simulink model "nn_fuel_control_4_15"  (R2021a)
settings: Solver=ode15s  StartTime=0.0  StopTime=T  MaxStep=.01  RelTol=1e-3
undefined symbols (not defined in the file): AF_sensor_tol, fault_time, fuel_inj_tol, kappa_tol, MAF_sensor_tol, pump_tol, tau_ww_tol
libraries: neural x66
(part 3 of 3)

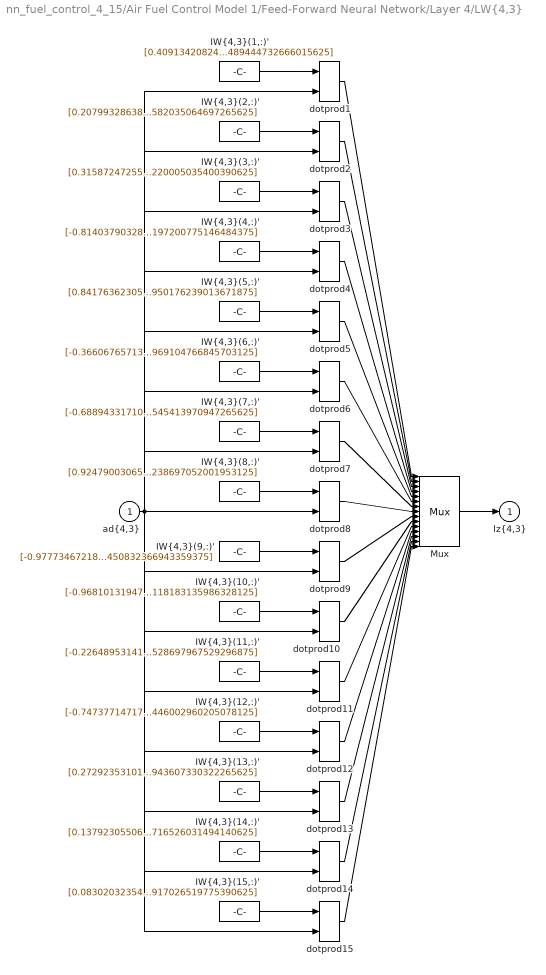
== system nn_fuel_control_4_15/Air Fuel Control Model 1/Feed-Forward Neural Network/Layer 4/LW{4,3} ==
  "ad{4,3}" : Inport  PortDimensions=15
      mask Display: e = 0.06;c1 = [120 230 180]/255;c2 = ([120 230 180]+0)/(256+128);c3 = ([120 230 180]+128)/(256+128);patch([0 1 1 0],[0 0 1 1],c1);patch([0 1 1 1-e 1-e 0+e],[0 0 1 1-e 0+e 0+e],c2);patch([0 0 1 1-e 0+e 0+e],[0 1 1 1-e 1-e 0+e],c3);plot([0 1 1 0 0],[0 0 1 1 0]);
  "IW{4,3}(1,:)'" : Constant  Value=[0.409134208241364427660613500847830437123775482177734375;-0.018608604712277689030575089645935804583132266998291015625;-0.429419328749681750156952375618857331573963165283203125;0.0968634595111320939597732149195508100092411041259765625;0.161200991521329939359929994679987430572509765625;-0.008332083953835521528130669821621268056333065032958984375;0.2000331787879461586943108386549283750355243682861328125;0.10950567443581950277664560644552693702280521392822265625;0.2065467508985891764705655759826186113059520721435546875;0.9045530959878378407523769055842421948909759521484375;0.0283070330066618157383029341644942178390920162200927734375;0.1527128132980928310047374907298944890499114990234375;0.57805498370952645981191153623512946069240570068359375;-0.493604151024888526677614208892919123172760009765625;0.29996514325046830240495410180301405489444732666015625]
      mask Display: e = 0.06;c1 = [120 150 230]/255;c2 = ([120 150 230]+0)/383;c3 = ([120 150 230]+128)/383;patch([0 1 1 0],[0 0 1 1],c1);patch([0 1 1 1-e 1-e 0+e],[0 0 1 1-e 0+e 0+e],c2);patch([0 0 1 1-e 0+e 0+e],[0 1 1 1-e 1-e 0+e],c3);plot([0 1 1 0 0],[0 0 1 1 0]);disp('weights');
  "IW{4,3}(10,:)'" : Constant  Value=[-0.9681013194700429647099326757597737014293670654296875;0.308531151003858639114696416072547435760498046875;0.5238840389262133800940546279889531433582305908203125;-0.8084989587128526000725514677469618618488311767578125;-0.801873444424249459672182638314552605152130126953125;0.142650764746548308625762047086027450859546661376953125;-0.63857819911989810446328874604660086333751678466796875;-0.174290199895392905471425137875485233962535858154296875;-0.34415160909336417471848790228250436484813690185546875;-0.6047578233492736377030496441875584423542022705078125;-0.5627993624805025518753609503619372844696044921875;0.2576274618067879718097401564591564238071441650390625;-0.12046847177087678659734848451989819295704364776611328125;0.7481637664193332426521010347642004489898681640625;0.71881850459924578888859514336218126118183135986328125]
      mask Display: e = 0.06;c1 = [120 150 230]/255;c2 = ([120 150 230]+0)/383;c3 = ([120 150 230]+128)/383;patch([0 1 1 0],[0 0 1 1],c1);patch([0 1 1 1-e 1-e 0+e],[0 0 1 1-e 0+e 0+e],c2);patch([0 0 1 1-e 0+e 0+e],[0 1 1 1-e 1-e 0+e],c3);plot([0 1 1 0 0],[0 0 1 1 0]);disp('weights');
  "IW{4,3}(11,:)'" : Constant  Value=[-0.22648953141163108426781036541797220706939697265625;-0.4126513309446071531283450894989073276519775390625;-0.919897514578432495824245052062906324863433837890625;-0.4049584327914892423194714865530841052532196044921875;-0.9260658560814845063902112087816931307315826416015625;0.247532816868120786324425353086553514003753662109375;-0.8130784976056506518915512060630135238170623779296875;-0.1161494390508523988359002032666467130184173583984375;0.76460872230926124615280059515498578548431396484375;0.530450464187323778020299869240261614322662353515625;-0.6035021468768022590012378714163787662982940673828125;0.0287139365740867180676332282018847763538360595703125;-0.2066484644619717148117388205719180405139923095703125;-0.5723818088758767519408365842537023127079010009765625;-0.5211382354194913357758878191816620528697967529296875]
      mask Display: e = 0.06;c1 = [120 150 230]/255;c2 = ([120 150 230]+0)/383;c3 = ([120 150 230]+128)/383;patch([0 1 1 0],[0 0 1 1],c1);patch([0 1 1 1-e 1-e 0+e],[0 0 1 1-e 0+e 0+e],c2);patch([0 0 1 1-e 0+e 0+e],[0 1 1 1-e 1-e 0+e],c3);plot([0 1 1 0 0],[0 0 1 1 0]);disp('weights');
  "IW{4,3}(12,:)'" : Constant  Value=[-0.747377147172722633428065819316543638706207275390625;-0.89961393161859748435205119676538743078708648681640625;-0.037086697665867023043784200808659079484641551971435546875;-0.5886496554696816208007703608018346130847930908203125;0.840702237392853657382829624111764132976531982421875;0.68778578029264991755553637631237506866455078125;-0.09030666083632643559298003310686908662319183349609375;0.5165108873683141865740253706462681293487548828125;-0.89460884910017035576146327002788893878459930419921875;-0.82058175976433034293222590349614620208740234375;0.6131893427537697949247785800253041088581085205078125;0.699855135033757402851506412844173610210418701171875;-0.335585846707859014603769765017204917967319488525390625;0.0423943456344091362808512712945230305194854736328125;0.297963040188151062626076281958376057446002960205078125]
      mask Display: e = 0.06;c1 = [120 150 230]/255;c2 = ([120 150 230]+0)/383;c3 = ([120 150 230]+128)/383;patch([0 1 1 0],[0 0 1 1],c1);patch([0 1 1 1-e 1-e 0+e],[0 0 1 1-e 0+e 0+e],c2);patch([0 0 1 1-e 0+e 0+e],[0 1 1 1-e 1-e 0+e],c3);plot([0 1 1 0 0],[0 0 1 1 0]);disp('weights');
  "IW{4,3}(13,:)'" : Constant  Value=[0.27292353101536026560580694422242231667041778564453125;0.291784885724885867386291238290141336619853973388671875;0.8796340464296978911562518987921066582202911376953125;0.307061729491277357606549003321561031043529510498046875;-0.3222728751950858505637143025523982942104339599609375;0.0304681963646269045320469359694470767863094806671142578125;-0.2456543422635725504310499900384456850588321685791015625;-0.89682596908113521028127479439717717468738555908203125;-0.28255076861598527049324047766276635229587554931640625;0.3030535285194508876571717337355948984622955322265625;-0.67415060674015503394684856175445020198822021484375;0.6670352766341516304038350426708348095417022705078125;0.2667146340046648855803823607857339084148406982421875;-0.045954538378264686571128549985587596893310546875;0.2340639218102315288749792898670420981943607330322265625]
      mask Display: e = 0.06;c1 = [120 150 230]/255;c2 = ([120 150 230]+0)/383;c3 = ([120 150 230]+128)/383;patch([0 1 1 0],[0 0 1 1],c1);patch([0 1 1 1-e 1-e 0+e],[0 0 1 1-e 0+e 0+e],c2);patch([0 0 1 1-e 0+e 0+e],[0 1 1 1-e 1-e 0+e],c3);plot([0 1 1 0 0],[0 0 1 1 0]);disp('weights');
  "IW{4,3}(14,:)'" : Constant  Value=[0.1379230550644596764442439962294884026050567626953125;0.4775263823187978484696714076562784612178802490234375;-0.006364787120916037821416466613300144672393798828125;0.43980447972305025672312694950960576534271240234375;-0.6384608804287079664163684356026351451873779296875;-0.03130848387336104821088156313635408878326416015625;0.9574895373112684016092543970444239675998687744140625;-0.0896234843262868619007122106268070638179779052734375;0.1527953241303305897957898196182213723659515380859375;-0.1292468261657202521774934211862273514270782470703125;-0.970451720093115977050501896883361041545867919921875;-0.165062170367600291598364492529071867465972900390625;-0.7332719341796412049205855510081164538860321044921875;0.15986676798598864479572512209415435791015625;-0.6782299146816017643146778937079943716526031494140625]
      mask Display: e = 0.06;c1 = [120 150 230]/255;c2 = ([120 150 230]+0)/383;c3 = ([120 150 230]+128)/383;patch([0 1 1 0],[0 0 1 1],c1);patch([0 1 1 1-e 1-e 0+e],[0 0 1 1-e 0+e 0+e],c2);patch([0 0 1 1-e 0+e 0+e],[0 1 1 1-e 1-e 0+e],c3);plot([0 1 1 0 0],[0 0 1 1 0]);disp('weights');
  "IW{4,3}(15,:)'" : Constant  Value=[0.08302032354421218229845180758275091648101806640625;0.249954151496840193402704244363121688365936279296875;0.5479301525869659794665267327218316495418548583984375;0.1693125052219013326748608960770070552825927734375;0.7569645787080911958355500246398150920867919921875;-0.8852503867351309008171256209607236087322235107421875;-0.6961185761680448447208391371532343327999114990234375;-0.5600757389611796810413579805754125118255615234375;-0.0720835330077151947847369228838942945003509521484375;0.855447974963159385453081995365209877490997314453125;0.167257696778575937202049317420460283756256103515625;-0.2562635879714936226747568071004934608936309814453125;-0.90062487978110539188492111861705780029296875;-0.11820475372601801922201048000715672969818115234375;-0.4539894984214323248039590907865203917026519775390625]
      mask Display: e = 0.06;c1 = [120 150 230]/255;c2 = ([120 150 230]+0)/383;c3 = ([120 150 230]+128)/383;patch([0 1 1 0],[0 0 1 1],c1);patch([0 1 1 1-e 1-e 0+e],[0 0 1 1-e 0+e 0+e],c2);patch([0 0 1 1-e 0+e 0+e],[0 1 1 1-e 1-e 0+e],c3);plot([0 1 1 0 0],[0 0 1 1 0]);disp('weights');
  "IW{4,3}(2,:)'" : Constant  Value=[0.2079932863873300286083889432120486162602901458740234375;0.0198375850467484675376805824953407864086329936981201171875;-0.0170538332699734680730774272205962915904819965362548828125;-0.78563968744001211330640899177524261176586151123046875;-0.2368930020652066925634926519705913960933685302734375;0.9350198499073567592887457067263312637805938720703125;-0.12408787305239055154260086055728606879711151123046875;0.405654658867162176694165509616141207516193389892578125;0.53267120540349510715572023400454781949520111083984375;0.2861429337433631925335930645815096795558929443359375;0.55828534790967221379531792990746907889842987060546875;0.1589999460246069862279227891121990978717803955078125;-0.67481637945571459891169752154382877051830291748046875;0.1334057042983116669887522220960818231105804443359375;0.7580972863172894538053014912293292582035064697265625]
      mask Display: e = 0.06;c1 = [120 150 230]/255;c2 = ([120 150 230]+0)/383;c3 = ([120 150 230]+128)/383;patch([0 1 1 0],[0 0 1 1],c1);patch([0 1 1 1-e 1-e 0+e],[0 0 1 1-e 0+e 0+e],c2);patch([0 0 1 1-e 0+e 0+e],[0 1 1 1-e 1-e 0+e],c3);plot([0 1 1 0 0],[0 0 1 1 0]);disp('weights');
  "IW{4,3}(3,:)'" : Constant  Value=[0.315872472556143424338159775288659147918224334716796875;0.1333374680748961316201217641719267703592777252197265625;-0.8918022391931847980828251820639707148075103759765625;0.7229899645184658663055188299040310084819793701171875;-0.2253949295409380937371679465286433696746826171875;0.43626032290268312863190658390522003173828125;-0.328908135182625349646201584619120694696903228759765625;-0.458606144094257428545091670457622967660427093505859375;-0.61397105979310195866816002308041788637638092041015625;0.687755868493051369938484640442766249179840087890625;-0.55032022765885801884877537304419092833995819091796875;-0.984145967069915972302851514541544020175933837890625;0.659406042092762323392207690631039440631866455078125;0.7727829791426754635352835975936613976955413818359375;-0.2628597007919442063439419143833220005035400390625]
      mask Display: e = 0.06;c1 = [120 150 230]/255;c2 = ([120 150 230]+0)/383;c3 = ([120 150 230]+128)/383;patch([0 1 1 0],[0 0 1 1],c1);patch([0 1 1 1-e 1-e 0+e],[0 0 1 1-e 0+e 0+e],c2);patch([0 0 1 1-e 0+e 0+e],[0 1 1 1-e 1-e 0+e],c3);plot([0 1 1 0 0],[0 0 1 1 0]);disp('weights');
  "IW{4,3}(4,:)'" : Constant  Value=[-0.814037903285731001545855178846977651119232177734375;0.1890950378764437445067159160316805355250835418701171875;0.136401296266547567004323582295910455286502838134765625;0.360474784994809394067516450377297587692737579345703125;0.5630045830298939790736767463386058807373046875;0.29464287473444394915844668503268621861934661865234375;-0.166389331488835556793759451466030441224575042724609375;-0.52974791348181538008788038496277295053005218505859375;0.6709267757531172104989991566981188952922821044921875;0.78215070403519337816078405012376606464385986328125;-0.3475888728410432282345254861866123974323272705078125;-0.05233329279450771309711853973567485809326171875;-0.30839028431399395646650418711942620575428009033203125;-0.7896972970706410688279675014200620353221893310546875;-0.17608840795251889943529022275470197200775146484375]
      mask Display: e = 0.06;c1 = [120 150 230]/255;c2 = ([120 150 230]+0)/383;c3 = ([120 150 230]+128)/383;patch([0 1 1 0],[0 0 1 1],c1);patch([0 1 1 1-e 1-e 0+e],[0 0 1 1-e 0+e 0+e],c2);patch([0 0 1 1-e 0+e 0+e],[0 1 1 1-e 1-e 0+e],c3);plot([0 1 1 0 0],[0 0 1 1 0]);disp('weights');
  "IW{4,3}(5,:)'" : Constant  Value=[0.84176362305803476004939511767588555812835693359375;0.2477725819719711619626423271256498992443084716796875;0.5861173758530409116929149604402482509613037109375;-0.2752688473484992126572024062625132501125335693359375;0.51232493805437240297351308981887996196746826171875;-0.617883791172630925103703702916391193866729736328125;0.0601814606396653406505947714322246611118316650390625;-0.407352526024439942631261146743781864643096923828125;-0.2072883860196756966587372517096810042858123779296875;-0.49975965526174181974283783347345888614654541015625;-0.40148233621736295617665746249258518218994140625;-0.852800606242346770358153662527911365032196044921875;-0.9196593002841557673576744491583667695522308349609375;0.2861473976537853847190717715420760214328765869140625;-0.1468670488112422400917012055288068950176239013671875]
      mask Display: e = 0.06;c1 = [120 150 230]/255;c2 = ([120 150 230]+0)/383;c3 = ([120 150 230]+128)/383;patch([0 1 1 0],[0 0 1 1],c1);patch([0 1 1 1-e 1-e 0+e],[0 0 1 1-e 0+e 0+e],c2);patch([0 0 1 1-e 0+e 0+e],[0 1 1 1-e 1-e 0+e],c3);plot([0 1 1 0 0],[0 0 1 1 0]);disp('weights');
  "IW{4,3}(6,:)'" : Constant  Value=[-0.366067657130750567784360782752628438174724578857421875;-0.5885259561877165257470778669812716543674468994140625;-0.73842489905764419066969139748835004866123199462890625;0.714576283962894631685003332677297294139862060546875;-0.0609476018705905620009843914886005222797393798828125;0.73355928402501680007929962812340818345546722412109375;0.1474523444056059506834799321950413286685943603515625;-0.2160830186712152656269836370483972132205963134765625;0.33658785604271823643784955493174493312835693359375;-0.6737160690455079592453557779663242399692535400390625;0.49385592210495332654573985564638860523700714111328125;-0.6063479899954280494256408928777091205120086669921875;0.6470220483020143742436403044848702847957611083984375;-0.205829216943276716023092376417480409145355224609375;-0.920350237519944158748330664820969104766845703125]
      mask Display: e = 0.06;c1 = [120 150 230]/255;c2 = ([120 150 230]+0)/383;c3 = ([120 150 230]+128)/383;patch([0 1 1 0],[0 0 1 1],c1);patch([0 1 1 1-e 1-e 0+e],[0 0 1 1-e 0+e 0+e],c2);patch([0 0 1 1-e 0+e 0+e],[0 1 1 1-e 1-e 0+e],c3);plot([0 1 1 0 0],[0 0 1 1 0]);disp('weights');
  "IW{4,3}(7,:)'" : Constant  Value=[-0.688943317105236818775892970734275877475738525390625;-0.5417308519282884038403835802455432713031768798828125;-0.2521322205228260227016789940535090863704681396484375;0.94374276814532809254387757391668856143951416015625;0.1889533323761056760048404612462036311626434326171875;-0.9318119687351316127177369708078913390636444091796875;0.4540745589147954230924142393632791936397552490234375;-0.5142256715696016389216538300388492643833160400390625;0.4877526756618586478708721188013441860675811767578125;-0.2884862767777562897464349589427001774311065673828125;0.3008932019526311396617757054627873003482818603515625;-0.089609771299732354776779175153933465480804443359375;0.5886547451838171074456340647884644567966461181640625;0.0935276670241786955983798179659061133861541748046875;-0.916953528583667409890267663286067545413970947265625]
      mask Display: e = 0.06;c1 = [120 150 230]/255;c2 = ([120 150 230]+0)/383;c3 = ([120 150 230]+128)/383;patch([0 1 1 0],[0 0 1 1],c1);patch([0 1 1 1-e 1-e 0+e],[0 0 1 1-e 0+e 0+e],c2);patch([0 0 1 1-e 0+e 0+e],[0 1 1 1-e 1-e 0+e],c3);plot([0 1 1 0 0],[0 0 1 1 0]);disp('weights');
  "IW{4,3}(8,:)'" : Constant  Value=[0.9247900306516465551709416104131378233432769775390625;-0.451872576203322662280470467521809041500091552734375;0.2144636938109696633336653803780791349709033966064453125;0.47393632788181161430429710890166461467742919921875;-0.5967841378403215824022254309966228902339935302734375;0.08921929855929823516280663397992611862719058990478515625;0.50281570056286717385063411711598746478557586669921875;-0.2361795031497051222668659420378389768302440643310546875;0.28420950093741248476675309575512073934078216552734375;-0.0425352900120927746030474736471660435199737548828125;0.393770417536720263029792477027513086795806884765625;0.6773406762422686799851589967147447168827056884765625;0.62704069904055137474330194891081191599369049072265625;0.0260862162785266971098963040276430547237396240234375;0.71691198886489904129604155968991108238697052001953125]
      mask Display: e = 0.06;c1 = [120 150 230]/255;c2 = ([120 150 230]+0)/383;c3 = ([120 150 230]+128)/383;patch([0 1 1 0],[0 0 1 1],c1);patch([0 1 1 1-e 1-e 0+e],[0 0 1 1-e 0+e 0+e],c2);patch([0 0 1 1-e 0+e 0+e],[0 1 1 1-e 1-e 0+e],c3);plot([0 1 1 0 0],[0 0 1 1 0]);disp('weights');
  "IW{4,3}(9,:)'" : Constant  Value=[-0.9777346721832860243495133545366115868091583251953125;0.3448850057379984068717249101609922945499420166015625;0.3117068047075581826987900058156810700893402099609375;-0.2800738720389521763109996754792518913745880126953125;0.1829551461951293145347108293208293616771697998046875;-0.036462488845966589678937452845275402069091796875;0.61637847324658689984744341927580535411834716796875;-0.97795607139009721464617541641928255558013916015625;-0.306381255697655507930221574497409164905548095703125;-0.3682386527599306180746907557477243244647979736328125;0.636545889474316783918084183824248611927032470703125;0.67733149686665061750545646646060049533843994140625;-0.1690740091796387734035533867427147924900054931640625;0.3344301037607857463029858990921638906002044677734375;-0.21065411005500944696677834144793450832366943359375]
      mask Display: e = 0.06;c1 = [120 150 230]/255;c2 = ([120 150 230]+0)/383;c3 = ([120 150 230]+128)/383;patch([0 1 1 0],[0 0 1 1],c1);patch([0 1 1 1-e 1-e 0+e],[0 0 1 1-e 0+e 0+e],c2);patch([0 0 1 1-e 0+e 0+e],[0 1 1 1-e 1-e 0+e],c3);plot([0 1 1 0 0],[0 0 1 1 0]);disp('weights');
  Mux : Mux  Inputs=15
      mask Display: e = 0.06;c1 = [120 150 230]/255;c2 = ([120 150 230]+0)/383;c3 = ([120 150 230]+128)/383;patch([0 1 1 0],[0 0 1 1],c1);patch([0 1 1 1-e 1-e 0+e],[0 0 1 1-e 0+e 0+e],c2);patch([0 0 1 1-e 0+e 0+e],[0 1 1 1-e 1-e 0+e],c3);plot([0 1 1 0 0],[0 0 1 1 0]);disp('Mux');
  dotprod{1..15} (15 alike) : neural/Weight Functions/dotprod
  "lz{4,3}" : Outport
      mask Display: e = 0.06;c1 = [120 230 180]/255;c2 = ([120 230 180]+0)/(256+128);c3 = ([120 230 180]+128)/(256+128);patch([0 1 1 0],[0 0 1 1],c1);patch([0 1 1 1-e 1-e 0+e],[0 0 1 1-e 0+e 0+e],c2);patch([0 0 1 1-e 0+e 0+e],[0 1 1 1-e 1-e 0+e],c3);plot([0 1 1 0 0],[0 0 1 1 0]);
  wires:
  "IW{4,3}(1,:)'"/1 -> dotprod1/1
  "ad{4,3}"/1 -> dotprod1/2, dotprod2/2, dotprod3/2, dotprod4/2, dotprod5/2, dotprod6/2, dotprod7/2, dotprod8/2, dotprod9/2, dotprod10/2, dotprod11/2, dotprod12/2, dotprod13/2, dotprod14/2, dotprod15/2
  dotprod1/1 -> Mux/1
  "IW{4,3}(2,:)'"/1 -> dotprod2/1
  dotprod2/1 -> Mux/2
  "IW{4,3}(3,:)'"/1 -> dotprod3/1
  dotprod3/1 -> Mux/3
  "IW{4,3}(4,:)'"/1 -> dotprod4/1
  dotprod4/1 -> Mux/4
  "IW{4,3}(5,:)'"/1 -> dotprod5/1
  dotprod5/1 -> Mux/5
  "IW{4,3}(6,:)'"/1 -> dotprod6/1
  dotprod6/1 -> Mux/6
  "IW{4,3}(7,:)'"/1 -> dotprod7/1
  dotprod7/1 -> Mux/7
  "IW{4,3}(8,:)'"/1 -> dotprod8/1
  dotprod8/1 -> Mux/8
  "IW{4,3}(9,:)'"/1 -> dotprod9/1
  dotprod9/1 -> Mux/9
  "IW{4,3}(10,:)'"/1 -> dotprod10/1
  dotprod10/1 -> Mux/10
  "IW{4,3}(11,:)'"/1 -> dotprod11/1
  dotprod11/1 -> Mux/11
  "IW{4,3}(12,:)'"/1 -> dotprod12/1
  dotprod12/1 -> Mux/12
  "IW{4,3}(13,:)'"/1 -> dotprod13/1
  dotprod13/1 -> Mux/13
  "IW{4,3}(14,:)'"/1 -> dotprod14/1
  dotprod14/1 -> Mux/14
  "IW{4,3}(15,:)'"/1 -> dotprod15/1
  dotprod15/1 -> Mux/15
  Mux/1 -> "lz{4,3}"/1

== system nn_fuel_control_4_15/Air Fuel Control Model 1/Feed-Forward Neural Network/Layer 5/Delays 1 ==
  "p{5}" : Inport  PortDimensions=15
      mask Display: e = 0.06;c1 = [120 230 180]/255;c2 = ([120 230 180]+0)/(256+128);c3 = ([120 230 180]+128)/(256+128);patch([0 1 1 0],[0 0 1 1],c1);patch([0 1 1 1-e 1-e 0+e],[0 0 1 1-e 0+e 0+e],c2);patch([0 0 1 1-e 0+e 0+e],[0 1 1 1-e 1-e 0+e],c3);plot([0 1 1 0 0],[0 0 1 1 0]);
  mux : Mux  Inputs=1
      mask Display: e = 0.06;c1 = [120 150 230]/255;c2 = ([120 150 230]+0)/383;c3 = ([120 150 230]+128)/383;patch([0 1 1 0],[0 0 1 1],c1);patch([0 1 1 1-e 1-e 0+e],[0 0 1 1-e 0+e 0+e],c2);patch([0 0 1 1-e 0+e 0+e],[0 1 1 1-e 1-e 0+e],c3);plot([0 1 1 0 0],[0 0 1 1 0]);disp('Mux')
  "pd{5,4}" : Outport
      mask Display: e = 0.06;c1 = [120 230 180]/255;c2 = ([120 230 180]+0)/(256+128);c3 = ([120 230 180]+128)/(256+128);patch([0 1 1 0],[0 0 1 1],c1);patch([0 1 1 1-e 1-e 0+e],[0 0 1 1-e 0+e 0+e],c2);patch([0 0 1 1-e 0+e 0+e],[0 1 1 1-e 1-e 0+e],c3);plot([0 1 1 0 0],[0 0 1 1 0]);
  wires:
  "p{5}"/1 -> mux/1
  mux/1 -> "pd{5,4}"/1

== system nn_fuel_control_4_15/Air Fuel Control Model 1/Feed-Forward Neural Network/Layer 5/LW{5,4} ==
  "ad{5,4}" : Inport  PortDimensions=15
      mask Display: e = 0.06;c1 = [120 230 180]/255;c2 = ([120 230 180]+0)/(256+128);c3 = ([120 230 180]+128)/(256+128);patch([0 1 1 0],[0 0 1 1],c1);patch([0 1 1 1-e 1-e 0+e],[0 0 1 1-e 0+e 0+e],c2);patch([0 0 1 1-e 0+e 0+e],[0 1 1 1-e 1-e 0+e],c3);plot([0 1 1 0 0],[0 0 1 1 0]);
  "IW{5,4}(1,:)'" : Constant  Value=[-0.76069441689470329581723717637942172586917877197265625;0.014695628439766288131362870217344607226550579071044921875;-0.5875265541395473523067494170391000807285308837890625;-0.8196023933676404027437456534244120121002197265625;0.9061263066130165189093759181560017168521881103515625;0.442303407245790036750321405634167604148387908935546875;-0.4886414939729564199666356216766871511936187744140625;-0.0870288732364914441319569959887303411960601806640625;0.755632847166979093600502892513759434223175048828125;0.2102185626740176449533947788950172252953052520751953125;0.5433839654741559055395327959558926522731781005859375;0.499494992315861530141063440169091336429119110107421875;-0.2189695297140807073166257623597630299627780914306640625;-0.268790265153092899907960600103251636028289794921875;0.50170101594177562986942575662396848201751708984375]
      mask Display: e = 0.06;c1 = [120 150 230]/255;c2 = ([120 150 230]+0)/383;c3 = ([120 150 230]+128)/383;patch([0 1 1 0],[0 0 1 1],c1);patch([0 1 1 1-e 1-e 0+e],[0 0 1 1-e 0+e 0+e],c2);patch([0 0 1 1-e 0+e 0+e],[0 1 1 1-e 1-e 0+e],c3);plot([0 1 1 0 0],[0 0 1 1 0]);disp('weights');
  Mux : Mux  Inputs=1
      mask Display: e = 0.06;c1 = [120 150 230]/255;c2 = ([120 150 230]+0)/383;c3 = ([120 150 230]+128)/383;patch([0 1 1 0],[0 0 1 1],c1);patch([0 1 1 1-e 1-e 0+e],[0 0 1 1-e 0+e 0+e],c2);patch([0 0 1 1-e 0+e 0+e],[0 1 1 1-e 1-e 0+e],c3);plot([0 1 1 0 0],[0 0 1 1 0]);disp('Mux');
  dotprod1 : neural/Weight Functions/dotprod
  "lz{5,4}" : Outport
      mask Display: e = 0.06;c1 = [120 230 180]/255;c2 = ([120 230 180]+0)/(256+128);c3 = ([120 230 180]+128)/(256+128);patch([0 1 1 0],[0 0 1 1],c1);patch([0 1 1 1-e 1-e 0+e],[0 0 1 1-e 0+e 0+e],c2);patch([0 0 1 1-e 0+e 0+e],[0 1 1 1-e 1-e 0+e],c3);plot([0 1 1 0 0],[0 0 1 1 0]);
  wires:
  "IW{5,4}(1,:)'"/1 -> dotprod1/1
  "ad{5,4}"/1 -> dotprod1/2
  dotprod1/1 -> Mux/1
  Mux/1 -> "lz{5,4}"/1
